simulink model "MPCsim"  (R2017b)
settings: Solver=VariableStepAuto  StartTime=0.0  StopTime=1  RelTol=1e-3
settings Model: Creator=Ecstasy  LastModifiedBy=Ecstasy

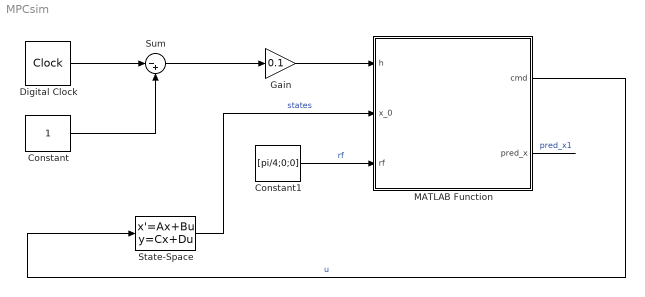
== system MPCsim ==
  Constant : Constant
  Constant1 : Constant  Value=[pi/4;0;0]
  Digital Clock : DigitalClock  SampleTime=0.001
  Gain : Gain  Gain=0.1
  MATLAB Function : MATLAB Function  TreatAsAtomicUnit=on
  State-Space : StateSpace  A=[0,1,0;0,0,1;0,0,0]  B=[0;0;1]  C=eye(3)  D=zeros(3,1)  InitialCondition=[0;0;0]
  Sum : Sum  Inputs=|-+
  wires:
  State-Space/1 -> MATLAB Function/2(x_0)  "states"
  MATLAB Function/1(cmd) -> State-Space/1  "u"
  Constant/1 -> Sum/2
  Digital Clock/1 -> Sum/1
  Sum/1 -> Gain/1
  Gain/1 -> MATLAB Function/1(h)
  Constant1/1 -> MATLAB Function/3(rf)  "rf"
  MATLAB Function/2(pred_x) -> ?  "pred_x1"

== matlab function MPCsim/MATLAB Function ==
  data: h input; cmd output; x_0 input; rf input; pred_x output
function [cmd,pred_x] = calculate_cmd(h,x_0,rf)
    params.A = [1 h h^2*0.5;0 1 h;0 0 1];
    params.B = [7*h^3/12;h^2;h];
    params.Gamma_1h = [h^3/24;h^2/6;h/2];
    params.Q = diag([0,1,1]);
    params.R = 0.001;
    params.x_max = [2.8973;2.6100;15.0];
    params.x_min = -[2.8973;2.6100;15.0];
    params.u_max = 7500;
    params.x_0 = x_0;
    params.rf = rf;
    coder.extrinsic('csolve');
    vars_x = cell(10,1);
    vars_u = cell(9,1);
    for i = 1:10
        vars_x{i} = zeros(3,1);
        if (i<=9)
            vars_u{i} = zeros(1,1);
        end
    end
    vars = struct('u_0',0,'u_1',0,'u_2',0,'u_3',0,'u_4',0,'u_5',0,'u_6',0,...
        'u_7',0,'u_8',0,'u_9',0,'x_1',zeros(3,1),'x_2',zeros(3,1),'x_3',zeros(3,1),...
        'x_4',zeros(3,1),'x_5',zeros(3,1),'x_6',zeros(3,1),'x_7',zeros(3,1),...
        'x_8',zeros(3,1),'x_9',zeros(3,1),'x_10',zeros(3,1),'z_0',zeros(3,1),'z_1',zeros(3,1),...
        'z_2',zeros(3,1),'z_3',zeros(3,1),'z_4',zeros(3,1),'z_5',zeros(3,1),...
        'z_6',zeros(3,1),'z_7',zeros(3,1),'z_8',zeros(3,1),'z_9',zeros(3,1),...
        'z_10',zeros(3,1),'u',{vars_u},'x',{vars_x},'z',{vars_x});
    status = struct('optval',0,'gap',0,'steps',0,'converged',0);
    [vars,status] = csolve(params);
    cmd = vars.u_0;
    pred_x = vars.x_1;
end
